simulink model "model_6DOF_V01"  (R2024b)
settings: Solver=VariableStepAuto  StartTime=0.0  StopTime=4  RelTol=1e-3
undefined symbols (not defined in the file or in its folder): p_RatGearFr_na, p_RatGearRe_na, p_RatSt_na, p_trackFr_m, p_trackRe_m, VEH
libraries: simulink x12, autolibutils x3, VUT_lib x3, sharedtransform x2, vehdynlibtire x2, CTRL x1, ESTS x1, INP x1, FUSI x1, OUT x1, vehdynlibeom x1, vehdynlibsuspension x1
(part 1 of 3)
settings Model: Creator=blatak  LastModifiedBy=jmbsp

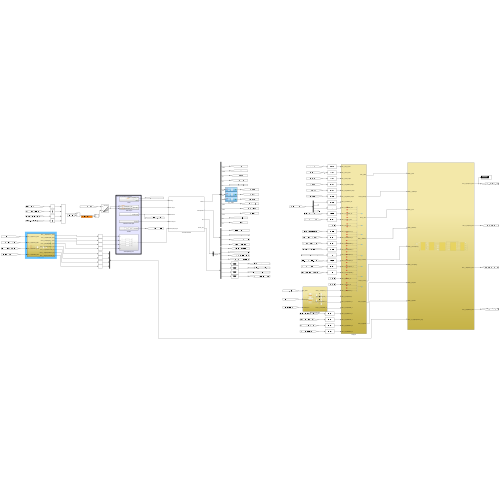
[thumbnail: Simulink's stored preview of the top-level diagram]
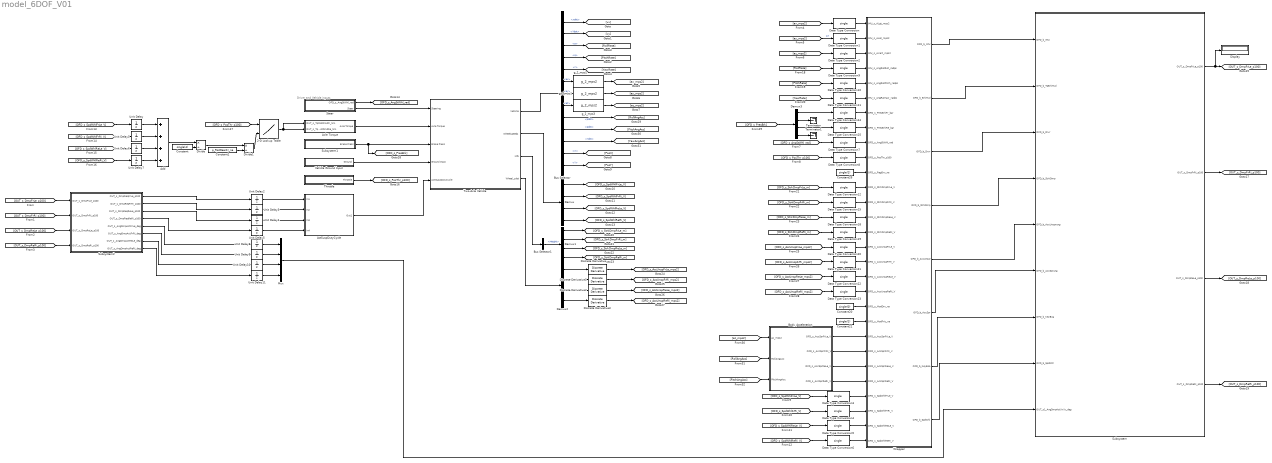
== system model_6DOF_V01 ==
  note: Driver and Vehicle inputs
  2-D Lookup Table : Lookup_n-D  BreakpointsForDimension1=[0 20 40 60 80 100]  BreakpointsForDimension2=[0 2000 4000 6000 8000 10000 12000]  Table=[0 0 0 0 0 0 0;200 200 200 200 150 100 50;350 350 350 250 200 150 100;500 500 500 350 250 150 150;650 650 650 450 350 250 200;800 800 800 600 500 400 300]  InternalRulePriority=Speed  RndMeth=Simplest
      settings: InputPortMap=u0,u1
  ActSuspDutyCycle : Subsystem
  Add : Sum  Inputs=++++
  Axle Torque : Subsystem
  Body_Acceleration : Subsystem
  Bus Selector : BusSelector  OutputSignals=Vehicle.BdyFrm.Cg.Vel.xdot,Vehicle.InertFrm.Cg.Vel.Ydot,Vehicle.BdyFrm.Cg.AngVel.p,Vehicle.BdyFrm.Cg.AngVel.q,Vehicle.BdyFrm.Cg.AngVel.r,Vehicle.BdyFrm.Cg.Acc.ax,Vehicle.BdyFrm.Cg.Acc.ay,Vehicle.BdyFrm.Cg.Acc.az,Vehicle.BdyFrm.Cg.AngAcc.pdot,Vehicle.BdyFrm.Cg.AngAcc.qdot,Vehicle.BdyFrm.Cg.AngAcc.rdot,Vehicle.InertFrm.Cg.Disp.X,Vehicle.InertFrm.Cg.Disp.Y
  Bus Selector1 : BusSelector  OutputSignals=Height
  Constant : Constant  Value=single(4)
  Constant1 : Constant  Value=p_RatGearFr_na
  Constant20 : Constant  Value=single(0)
  Constant21 : Constant  Value=single(1)
  Constant26 : Constant  Value=single(1)
  Data Type Conversion{,1..12,15,18..25} (22 alike) : DataTypeConversion  OutDataTypeStr=single  SaturateOnIntegerOverflow=off  RndMeth=Floor
  Demux{,1..3} (4 alike) : Demux
  Discrete Derivative{,1..3} (4 alike) : simulink/Discrete/Discrete Derivative  gainval=1.0  ICPrevScaledInput=0.0  OutMin=[]  OutMax=[]  OutDataType=fixdt(1, 16)  OutScaling=2^-10  DoSatur=off
  Display : Display
  Divide : Product  Inputs=*/
  Divide1 : Product  Inputs=*/
  Mux : Mux
  Steer : Subsystem
  Subsystem : Subsystem
  Subsystem1 : Subsystem
  Subsystem2 : Subsystem
  Terminator : Terminator
  Terminator1 : Terminator
  Throttle : Subsystem
  Two-Axle Vehicle : Subsystem
  Unit Delay{,1..11} (12 alike) : UnitDelay  SampleTime=-1  HasFrameUpgradeWarning=on
  Vehicle Ground Input : Subsystem  VariantControl=0
  Wrapper : Subsystem
  g_2_mps1 : VUT_lib/g_2_mps2  SystemSampleTime=-1  VariantActivationTime=update diagram  AllowFlexibleInterface=on  Latency=0  AutoFrameSizeCalculation=off
  g_2_mps2 : VUT_lib/g_2_mps2  SystemSampleTime=-1  VariantActivationTime=update diagram  AllowFlexibleInterface=on  Latency=0  AutoFrameSizeCalculation=off
  g_2_mps3 : VUT_lib/g_2_mps2  SystemSampleTime=-1  VariantActivationTime=update diagram  AllowFlexibleInterface=on  Latency=0  AutoFrameSizeCalculation=off
  wires:
  [OFD_s_AccUnspFrRi_mps2] -> Data Type Conversion21/1
  [OFD_s_AccUnspFrLe_mps2] -> Data Type Conversion20/1
  Data Type Conversion9/1 -> Wrapper/4(IMU_s_AngRatRoll_radps)
  Subsystem/1(OUT_s_DmpFrLe_p100) -> Display/1, [OUT_s_DmpFrLe_p100]
  Wrapper/7(OFD_b_KeyBoa) -> Subsystem/7(OFD_b_KeyBoa)
  Body_Acceleration/4(OFD_s_AccSprReRi_V) -> Wrapper/25(OFD_s_AccSprReRi_V)
  Body_Acceleration/1(OFD_s_AccSprFrLe_V) -> Wrapper/22(OFD_s_AccSprFrLe_V)
  Constant26/1 -> Wrapper/11(OFD_s_RegDrv_na)
  [ax_mps2] -> Data Type Conversion/1
  [OFD_s_AngStWhl_rad] -> Data Type Conversion7/1
  Body_Acceleration/2(OFD_s_AccSprFrRi_V) -> Wrapper/23(OFD_s_AccSprFrRi_V)
  Wrapper/1(OFD_b_IMU) -> Subsystem/1(OFD_b_IMU)
  [OFD_s_AccUnspReRi_mps2] -> Data Type Conversion23/1
  Constant20/1 -> Wrapper/20(OFD_s_ModDrv_na)
  [OFD_s_SpdWhlReRi_V] -> Data Type Conversion6/1
  Wrapper/8(OFD_b_SpdWhl) -> Subsystem/8(OFD_b_SpdWhl)
  Wrapper/4(OFD_b_StrkDmp) -> Subsystem/4(OFD_b_StrkDmp)
  Wrapper/2(OFD_b_BrkHyd) -> Subsystem/2(OFD_b_TqBrkHyd)
  [ay_mps2] -> Data Type Conversion1/1  "AY"
  [OFD_s_StrkDmpFrRi_m] -> Data Type Conversion15/1
  [OFD_s_StrkDmpReLe_m] -> Data Type Conversion18/1
  Wrapper/3(OFD_b_Drvr) -> Subsystem/3(OFD_b_Drvr)
  [OFD_s_AccUnspReLe_mps2] -> Data Type Conversion22/1
  [az_mps2] -> Data Type Conversion2/1
  Data Type Conversion10/1 -> Wrapper/5(IMU_s_AngRatPitch_radps)
  Wrapper/6(OFD_b_AccSpr) -> Subsystem/6(OFD_b_AccSprung)
  [OFD_s_SpdWhlReLe_V] -> Data Type Conversion5/1
  [OFD_s_StrkDmpReRi_m] -> Data Type Conversion19/1
  Demux3/1 -> Data Type Conversion24/1
  Subsystem/2(OUT_s_DmpFrRi_p100) -> [OUT_s_DmpFrRi_p100]
  Constant21/1 -> Wrapper/21(OFD_s_ModFric_na)
  [OFD_s_PosThr_p100] -> Data Type Conversion8/1
  Body_Acceleration/3(OFD_s_AccSprReLe_V) -> Wrapper/24(OFD_s_AccSprReLe_V)
  Wrapper/5(OFD_b_AccUnspr) -> Subsystem/5(OFD_b_AccUnsprung)
  Demux3/3 -> Data Type Conversion25/1
  [OFD_s_SpdWhlFrRi_V] -> Data Type Conversion4/1
  Data Type Conversion11/1 -> Wrapper/6(IMU_s_AngRatYaw_radps)
  [OFD_s_SpdWhlFrLe_V] -> Data Type Conversion3/1
  Subsystem/3(OUT_s_DmpReLe_p100) -> [OUT_s_DmpReLe_p100]
  g_2_mps2/1 -> [ax_mps2]
  Bus Selector/12 -> [PosX]  "<X>"
  Bus Selector/1 -> [vx]  "<xdot>"
  Throttle/1(Throttle) -> [OFD_s_PosThr_p100]
  Two-Axle Vehicle/1(Vehicle) -> Bus Selector/1
  Axle Torque/1(Axle Torque) -> Two-Axle Vehicle/2(Axle Torque)
  Bus Selector/13 -> [PosY]  "<Y>"
  Demux/2 -> [OFD_s_SpdWhlFrRi_V]
  Bus Selector/3 -> [RollRate]  "<p>"
  Demux/1 -> [OFD_s_SpdWhlFrLe_V]
  Bus Selector/5 -> [YawRate]  "<r>"
  g_2_mps1/1 -> [ay_mps2]
  Two-Axle Vehicle/2(Wheelspeeds) -> Demux/1
  2-D Lookup Table/1 -> Axle Torque/1(OUT_s_TqMotDmdFr_Nm), Axle Torque/2(OUT_s_TqMotDmdRe_Nm)
  Steer/1(OFD_s_AngStWhl_rad) -> [OFD_s_AngStWhl_rad]
  Vehicle Ground Input/1(Ground) -> Two-Axle Vehicle/4(Ground Input)
  Bus Selector/8 -> g_2_mps3/1  "<az>"
  g_2_mps3/1 -> [az_mps2]
  Bus Selector/6 -> g_2_mps2/1  "<ax>"
  Steer/2(Steer) -> Two-Axle Vehicle/1(Steering)
  Bus Selector/4 -> [PitchRate]  "<q>"
  Demux/3 -> [OFD_s_SpdWhlReLe_V]
  Demux/4 -> [OFD_s_SpdWhlReRi_V]
  Bus Selector/7 -> g_2_mps1/1  "<ay>"
  Bus Selector/2 -> [vy]  "<Ydot>"
  ActSuspDutyCycle/1(Out1) -> Two-Axle Vehicle/5(ActSuspDutyCycle)
  Unit Delay2/1 -> ActSuspDutyCycle/1(In1)
  Unit Delay3/1 -> ActSuspDutyCycle/2(In2)
  Unit Delay4/1 -> ActSuspDutyCycle/3(In3)
  Unit Delay5/1 -> ActSuspDutyCycle/4(In4)
  Subsystem/4(OUT_s_DmpReRi_p100) -> [OUT_s_DmpReRi_p100]
  Subsystem2/4(OUT_s_DmpReqReRi_p100) -> Unit Delay5/1
  Subsystem2/3(OUT_s_DmpReqReLe_p100) -> Unit Delay4/1
  Subsystem2/2(OUT_s_DmpReqFrRi_p100) -> Unit Delay3/1
  Subsystem2/1(OUT_s_DmpReqFrLe_p100) -> Unit Delay2/1
  Data Type Conversion/1 -> Wrapper/1(IMU_s_ALgt_mps2)
  Data Type Conversion1/1 -> Wrapper/2(IMU_s_ALat_mps2)
  Data Type Conversion2/1 -> Wrapper/3(IMU_s_AVert_mps2)
  Two-Axle Vehicle/3(Info) -> Bus Selector1/1
  Bus Selector1/1 -> Demux1/1  "<Height>"
  Data Type Conversion3/1 -> Wrapper/26(OFD_s_SpdWhlFrLe_V)
  Data Type Conversion4/1 -> Wrapper/27(OFD_s_SpdWhlFrRi_V)
  Data Type Conversion5/1 -> Wrapper/28(OFD_s_SpdWhlReLe_V)
  Data Type Conversion6/1 -> Wrapper/29(OFD_s_SpdWhlReRi_V)
  Data Type Conversion7/1 -> Wrapper/9(OFD_s_AngStWhl_rad)
  Data Type Conversion8/1 -> Wrapper/10(OFD_s_PosThr_p100)
  [OFD_s_SpdWhlFrLe_V] -> Unit Delay/1
  [OFD_s_SpdWhlFrRi_V] -> Unit Delay1/1
  [OFD_s_SpdWhlReLe_V] -> Unit Delay6/1
  [OFD_s_SpdWhlReRi_V] -> Unit Delay7/1
  Add/1 -> Divide/1
  Constant/1 -> Divide/2
  Divide/1 -> Divide1/1
  Constant1/1 -> Divide1/2
  Divide1/1 -> 2-D Lookup Table/2
  [OFD_s_PosThr_p100] -> 2-D Lookup Table/1
  Unit Delay/1 -> Add/1
  Unit Delay1/1 -> Add/2
  Unit Delay6/1 -> Add/3
  Unit Delay7/1 -> Add/4
  [RollRate] -> Data Type Conversion9/1
  [PitchRate] -> Data Type Conversion10/1
  [YawRate] -> Data Type Conversion11/1
  Demux1/1 -> [OFD_s_StrkDmpFrLe_m]
  Demux1/4 -> [OFD_s_StrkDmpReRi_m]
  Demux1/3 -> [OFD_s_StrkDmpReLe_m]
  Demux1/2 -> [OFD_s_StrkDmpFrRi_m]
  [OFD_s_StrkDmpFrLe_m] -> Data Type Conversion12/1
  Data Type Conversion12/1 -> Wrapper/12(OFD_s_StrkDmpFrLe_V)
  Data Type Conversion15/1 -> Wrapper/13(OFD_s_StrkDmpFrRi_V)
  Data Type Conversion18/1 -> Wrapper/14(OFD_s_StrkDmpReLe_V)
  Data Type Conversion19/1 -> Wrapper/15(OFD_s_StrkDmpReRi_V)
  Two-Axle Vehicle/4(Wheel_zdot) -> Demux2/1
  Demux2/1 -> Discrete Derivative/1
  Demux2/4 -> Discrete Derivative3/1
  Demux2/3 -> Discrete Derivative2/1
  Demux2/2 -> Discrete Derivative1/1
  Data Type Conversion20/1 -> Wrapper/16(OFD_s_AccUnspFrLe_V)
  Data Type Conversion21/1 -> Wrapper/17(OFD_s_AccUnspFrRi_V)
  Data Type Conversion22/1 -> Wrapper/18(OFD_s_AccUnspReLe_V)
  Data Type Conversion23/1 -> Wrapper/19(OFD_s_AccUnspReRi_V)
  [OFD_s_PresBrk] -> Demux3/1
  Demux3/2 -> Terminator/1
  Demux3/4 -> Terminator1/1
  Data Type Conversion24/1 -> Wrapper/7(OFD_s_PresBrkFr_bar)
  Data Type Conversion25/1 -> Wrapper/8(OFD_s_PresBrkRe_bar)
  Subsystem1/1(Brake Press) -> [OFD_s_PresBrk], Two-Axle Vehicle/3(Brake Press)
  Discrete Derivative/1 -> [OFD_s_AccUnspFrLe_mps2]
  Discrete Derivative1/1 -> [OFD_s_AccUnspFrRi_mps2]
  Discrete Derivative2/1 -> [OFD_s_AccUnspReLe_mps2]
  Discrete Derivative3/1 -> [OFD_s_AccUnspReRi_mps2]
  Bus Selector/9 -> [RollAngAcc]  "<pdot>"
  Bus Selector/10 -> [PitchAngAcc]  "<qdot>"
  Bus Selector/11 -> [YawAngAcc]  "<rdot>"
  [az_mps2] -> Body_Acceleration/1(az_mps2)
  [RollAngAcc] -> Body_Acceleration/2(RollAngAcc)
  [PitchAngAcc] -> Body_Acceleration/3(PitchAngAcc)
  [OUT_s_DmpFrLe_p100] -> Subsystem2/1(OUT_s_DmpFrLe_p100)
  [OUT_s_DmpFrRi_p100] -> Subsystem2/2(OUT_s_DmpFrRi_p100)
  [OUT_s_DmpReLe_p100] -> Subsystem2/3(OUT_s_DmpReLe_p100)
  [OUT_s_DmpReRi_p100] -> Subsystem2/4(OUT_s_DmpReRi_p100)
  Subsystem2/5(OUT_s_AngDmpActFrLe_deg) -> Unit Delay8/1
  Subsystem2/6(OUT_s_AngDmpActFrRi_deg) -> Unit Delay9/1
  Subsystem2/7(OUT_s_AngDmpActReLe_deg) -> Unit Delay10/1
  Subsystem2/8(OUT_s_AngDmpActReRi_deg) -> Unit Delay11/1
  Unit Delay11/1 -> Mux/4
  Unit Delay10/1 -> Mux/3
  Unit Delay9/1 -> Mux/2
  Unit Delay8/1 -> Mux/1
  Mux/1 -> Subsystem/9(OUT_s1_AngDmpActXxYy_deg)

== system model_6DOF_V01/ActSuspDutyCycle ==
  In1 : Inport
  In2 : Inport  Port=2
  In3 : Inport  Port=3
  In4 : Inport  Port=4
  Data Type Conversion{,1..3} (4 alike) : DataTypeConversion  OutDataTypeStr=double  SaturateOnIntegerOverflow=off  RndMeth=Floor
  Mux : Mux
  Out1 : Outport
  wires:
  Mux/1 -> Out1/1
  In1/1 -> Data Type Conversion/1
  Data Type Conversion/1 -> Mux/1
  In2/1 -> Data Type Conversion1/1
  Data Type Conversion1/1 -> Mux/2
  In3/1 -> Data Type Conversion2/1
  Data Type Conversion2/1 -> Mux/3
  In4/1 -> Data Type Conversion3/1
  Data Type Conversion3/1 -> Mux/4

== system model_6DOF_V01/Axle Torque ==
  OUT_s_TqMotDmdFr_Nm : Inport
  OUT_s_TqMotDmdRe_Nm : Inport  Port=2
  Constant1 : Constant  Value=p_RatGearRe_na
  Constant12 : Constant  Value=single(2)
  Constant2 : Constant  Value=single(2)
  Constant3 : Constant  Value=p_RatGearFr_na
  Data Type Conversion{,1..3} (4 alike) : DataTypeConversion  OutDataTypeStr=double  SaturateOnIntegerOverflow=off  RndMeth=Floor
  Divide : Product  Inputs=*/
  Divide1 : Product  Inputs=*/
  Mux : Mux
  Product : Product
  Product1 : Product
  Axle Torque : Outport
  wires:
  Mux/1 -> Axle Torque/1
  OUT_s_TqMotDmdFr_Nm/1 -> Product/2
  OUT_s_TqMotDmdRe_Nm/1 -> Product1/1
  Constant3/1 -> Product/1
  Constant1/1 -> Product1/2
  Product/1 -> Divide/1
  Constant12/1 -> Divide/2
  Product1/1 -> Divide1/1
  Constant2/1 -> Divide1/2
  Divide/1 -> Data Type Conversion1/1, Data Type Conversion/1
  Data Type Conversion/1 -> Mux/1
  Data Type Conversion1/1 -> Mux/2
  Data Type Conversion3/1 -> Mux/4
  Data Type Conversion2/1 -> Mux/3
  Divide1/1 -> Data Type Conversion3/1, Data Type Conversion2/1

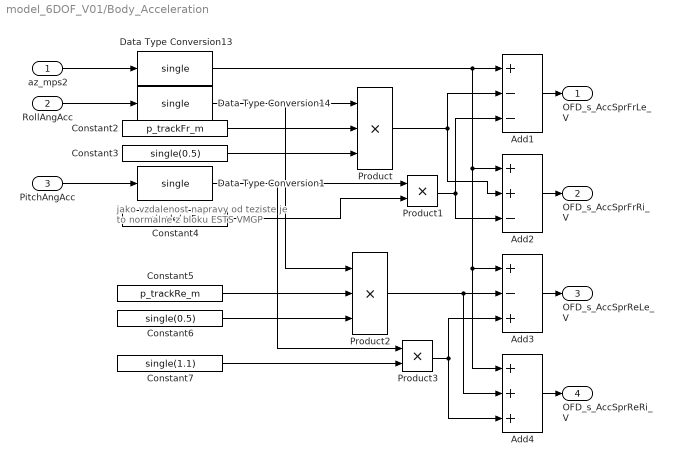
== system model_6DOF_V01/Body_Acceleration ==
  note: jako vzdalenost napravy od teziste
      | je to normalne z bloku ESTS VMGP
  az_mps2 : Inport
  RollAngAcc : Inport  Port=2
  PitchAngAcc : Inport  Port=3
  Add1 : Sum  Inputs=+--
  Add2 : Sum  Inputs=++-
  Add3 : Sum  Inputs=+-+
  Add4 : Sum  Inputs=+++
  Constant2 : Constant  Value=p_trackFr_m
  Constant3 : Constant  Value=single(0.5)
  Constant4 : Constant  Value=single(1.5)
  Constant5 : Constant  Value=p_trackRe_m
  Constant6 : Constant  Value=single(0.5)
  Constant7 : Constant  Value=single(1.1)
  Data Type Conversion1 : DataTypeConversion  OutDataTypeStr=single  SaturateOnIntegerOverflow=off  RndMeth=Floor
  Data Type Conversion13 : DataTypeConversion  OutDataTypeStr=single  SaturateOnIntegerOverflow=off  RndMeth=Floor
  Data Type Conversion14 : DataTypeConversion  OutDataTypeStr=single  SaturateOnIntegerOverflow=off  RndMeth=Floor
  Product : Product  Inputs=3
  Product1 : Product
  Product2 : Product  Inputs=3
  Product3 : Product
  OFD_s_AccSprFrLe_V : Outport
  OFD_s_AccSprFrRi_V : Outport  Port=2
  OFD_s_AccSprReLe_V : Outport  Port=3
  OFD_s_AccSprReRi_V : Outport  Port=4
  wires:
  Add3/1 -> OFD_s_AccSprReLe_V/1
  PitchAngAcc/1 -> Data Type Conversion1/1
  Product1/1 -> Add1/3, Add2/3
  Add1/1 -> OFD_s_AccSprFrLe_V/1
  Product2/1 -> Add4/2, Add3/2
  Data Type Conversion13/1 -> Add1/1, Add4/1, Add3/1, Add2/1
  Constant4/1 -> Product1/2
  Product/1 -> Add1/2, Add2/2
  Constant3/1 -> Product/3
  Constant7/1 -> Product3/2
  az_mps2/1 -> Data Type Conversion13/1
  Constant5/1 -> Product2/2
  Constant2/1 -> Product/2
  Product3/1 -> Add3/3, Add4/3
  Constant6/1 -> Product2/3
  Add4/1 -> OFD_s_AccSprReRi_V/1
  Add2/1 -> OFD_s_AccSprFrRi_V/1
  RollAngAcc/1 -> Data Type Conversion14/1
  Data Type Conversion1/1 -> Product3/1, Product1/1
  Data Type Conversion14/1 -> Product2/1, Product/1

== system model_6DOF_V01/Steer ==
  Constant22 : Constant  Value=p_RatSt_na
  Divide : Product  Inputs=*/
  Mux : Mux  Inputs=2
  Ramp : simulink/Sources/Ramp  slope=0.5  start=2  InitialOutput=0
  Saturation : Saturate  UpperLimit=1  LowerLimit=-1
  OFD_s_AngStWhl_rad : Outport
  Steer : Outport  Port=2
  wires:
  Mux/1 -> Steer/1
  Saturation/1 -> OFD_s_AngStWhl_rad/1, Divide/1
  Constant22/1 -> Divide/2
  Divide/1 -> Mux/2, Mux/1  "WhlStAng"
  Ramp/1 -> Saturation/1

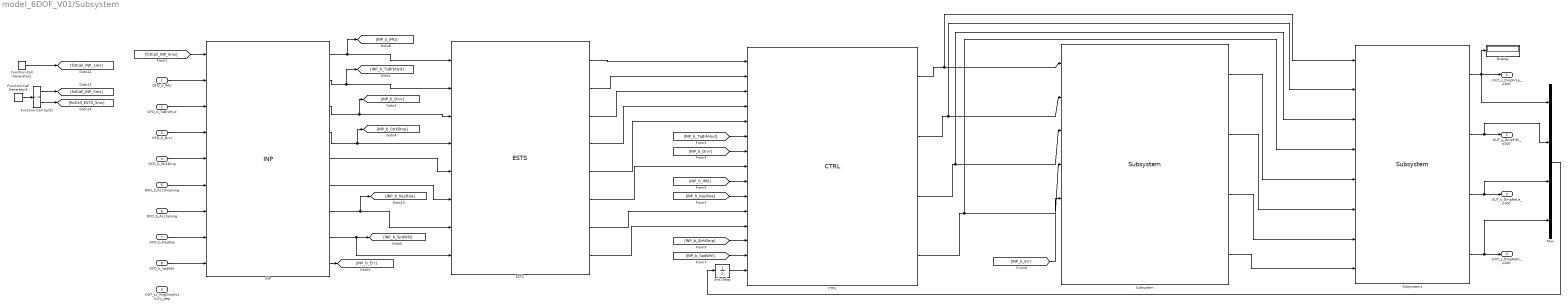
== system model_6DOF_V01/Subsystem ==
  OFD_b_IMU : Inport
  OFD_b_TqBrkHyd : Inport  Port=2
  OFD_b_Drvr : Inport  Port=3
  OFD_b_StrkDmp : Inport  Port=4
  OFD_b_AccUnsprung : Inport  Port=5
  OFD_b_AccSprung : Inport  Port=6
  OFD_b_KeyBoa : Inport  Port=7
  OFD_b_SpdWhl : Inport  Port=8
  OUT_s1_AngDmpActXxYy_deg : Inport  Port=9
  CTRL : CTRL/CTRL  SystemSampleTime=-1  VariantActivationTime=update diagram  AllowFlexibleInterface=on  Latency=0  AutoFrameSizeCalculation=off
  Display : Display
  ESTS : ESTS/ESTS  SystemSampleTime=-1  VariantActivationTime=update diagram  AllowFlexibleInterface=on  Latency=0  AutoFrameSizeCalculation=off
  Function-Call Generator2 : simulink/Ports & Subsystems/Function-Call Generator  sample_time=1  numberOfIterations=1  DisallowWideOutput=off
  Function-Call Generator3 : simulink/Ports & Subsystems/Function-Call Generator  sample_time=0.005  numberOfIterations=1  DisallowWideOutput=off
  Function-Call Split1 : FunctionCallSplit  IconShape=distinctive  NumOutputPorts=2  OutputPortLayout=default
  INP : INP/INP  SystemSampleTime=-1  VariantActivationTime=update diagram  AllowFlexibleInterface=on  Latency=0  AutoFrameSizeCalculation=off
      link override Function-Call Subsystem1/Bus Selector2: OutputSignals=OFD_s_AngStWhl_rad,OFD_s_PosThr_p100,OFD_s_RegDrv_na
  Mux : Mux
  Subsystem : FUSI/Subsystem  SystemSampleTime=-1  VariantActivationTime=update diagram  AllowFlexibleInterface=on  Latency=0  AutoFrameSizeCalculation=off
  Subsystem1 : OUT/Subsystem  SystemSampleTime=-1  VariantActivationTime=update diagram  AllowFlexibleInterface=on  Latency=0  AutoFrameSizeCalculation=off
  Unit Delay : UnitDelay  SampleTime=-1  HasFrameUpgradeWarning=on
  OUT_s_DmpFrLe_p100 : Outport
  OUT_s_DmpFrRi_p100 : Outport  Port=2
  OUT_s_DmpReLe_p100 : Outport  Port=3
  OUT_s_DmpReRi_p100 : Outport  Port=4
  wires:
  OFD_b_IMU/1 -> INP/2
  [fctCall_INP_5ms] -> INP/1
  OFD_b_Drvr/1 -> INP/4
  INP/3 -> [INP_b_Drvr], ESTS/3
  Function-Call Generator2/1 -> [fctCall_INP_1ms]
  Function-Call Generator3/1 -> Function-Call Split1/1
  INP/1 -> ESTS/1, [INP_b_IMU]
  Function-Call Split1/1 -> [fctCall_INP_5ms]
  Function-Call Split1/2 -> [fctCall_ESTS_5ms]
  ESTS/7 -> CTRL/11
  [INP_b_KeyBoa] -> CTRL/10
  [INP_b_Drvr] -> CTRL/7
  [INP_b_TqBrkHyd] -> CTRL/6
  ESTS/6 -> CTRL/8
  [INP_b_IMU] -> CTRL/9
  CTRL/1 -> Subsystem1/1, Subsystem/1
  CTRL/2 -> Subsystem1/2, Subsystem/2
  CTRL/3 -> Subsystem1/3, Subsystem/3
  CTRL/4 -> Subsystem1/4, Subsystem/4
  Subsystem1/1 -> Display/1, Mux/1, OUT_s_DmpFrLe_p100/1
  Subsystem1/2 -> Mux/2, OUT_s_DmpFrRi_p100/1
  Subsystem1/3 -> Mux/3, OUT_s_DmpReLe_p100/1
  Subsystem1/4 -> Mux/4, OUT_s_DmpReRi_p100/1
  [INP_b_StrkDmp] -> CTRL/13
  OFD_b_TqBrkHyd/1 -> INP/3
  OFD_b_StrkDmp/1 -> INP/5
  OFD_b_AccUnsprung/1 -> INP/6
  OFD_b_AccSprung/1 -> INP/7
  OFD_b_KeyBoa/1 -> INP/8
  INP/2 -> ESTS/2, [INP_b_TqBrkHyd]
  INP/4 -> [INP_b_StrkDmp], ESTS/4
  INP/5 -> ESTS/5
  INP/6 -> ESTS/6
  INP/7 -> ESTS/7, [INP_b_KeyBoa]
  ESTS/1 -> CTRL/1
  ESTS/2 -> CTRL/2
  ESTS/3 -> CTRL/3
  ESTS/4 -> CTRL/4
  ESTS/5 -> CTRL/5
  ESTS/8 -> CTRL/12
  [INP_b_Err] -> Subsystem/5
  Subsystem/1 -> Subsystem1/5
  Subsystem/2 -> Subsystem1/6
  Subsystem/3 -> Subsystem1/7
  Subsystem/4 -> Subsystem1/8
  OFD_b_SpdWhl/1 -> INP/9
  INP/8 -> [INP_b_SpdWhl], ESTS/8
  INP/9 -> [INP_b_Err]
  [INP_b_SpdWhl] -> CTRL/14
  Mux/1 -> Unit Delay/1
  Unit Delay/1 -> CTRL/15

== system model_6DOF_V01/Subsystem1 ==
  Mux : Mux
  Ramp : simulink/Sources/Ramp  slope=0  start=0  InitialOutput=0
  Saturation : Saturate
  Brake Press : Outport
  wires:
  Saturation/1 -> Mux/4, Mux/3, Mux/2, Mux/1
  Ramp/1 -> Saturation/1
  Mux/1 -> Brake Press/1

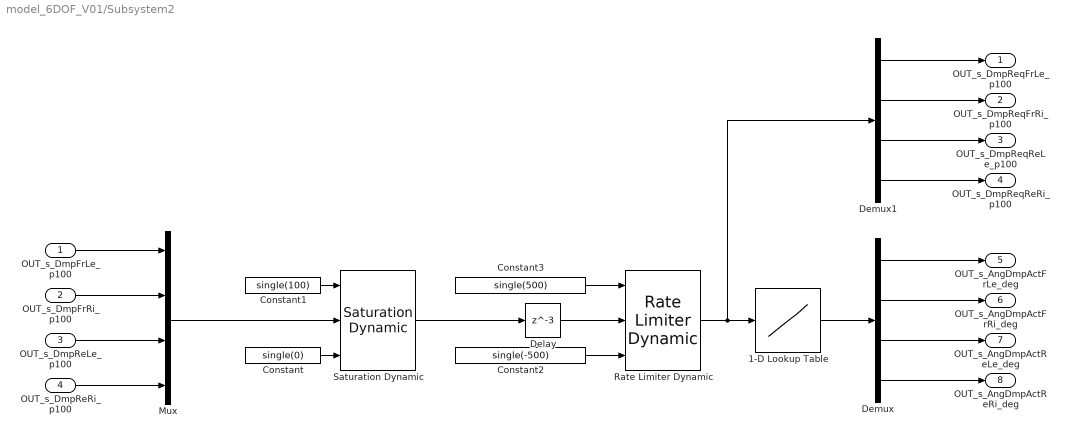
== system model_6DOF_V01/Subsystem2 ==
  OUT_s_DmpFrLe_p100 : Inport
  OUT_s_DmpFrRi_p100 : Inport  Port=2
  OUT_s_DmpReLe_p100 : Inport  Port=3
  OUT_s_DmpReRi_p100 : Inport  Port=4
  1-D Lookup Table : Lookup_n-D  NumberOfTableDimensions=1  BreakpointsForDimension1=[0 10 20 30 40 50 60 70 80 90 100]  Table=[0 5 10 15 20 25 30 35 40 45 50]  InternalRulePriority=Speed  RndMeth=Simplest
  Constant : Constant  Value=single(0)
  Constant1 : Constant  Value=single(100)
  Constant2 : Constant  Value=single(-500)
  Constant3 : Constant  Value=single(500)
  Delay : Delay  DelayLength=3
  Demux : Demux
  Demux1 : Demux
  Mux : Mux
  Rate Limiter Dynamic : simulink/Discontinuities/Rate Limiter Dynamic
  Saturation Dynamic : simulink/Discontinuities/Saturation Dynamic  OutMin=[]  OutMax=[]  OutDataTypeStr=Inherit: Same as second input  OutDataType=fixdt(1, 16)  OutScaling=2^-10  DoSatur=off
  OUT_s_DmpReqFrLe_p100 : Outport
  OUT_s_DmpReqFrRi_p100 : Outport  Port=2
  OUT_s_DmpReqReLe_p100 : Outport  Port=3
  OUT_s_DmpReqReRi_p100 : Outport  Port=4
  OUT_s_AngDmpActFrLe_deg : Outport  Port=5
  OUT_s_AngDmpActFrRi_deg : Outport  Port=6
  OUT_s_AngDmpActReLe_deg : Outport  Port=7
  OUT_s_AngDmpActReRi_deg : Outport  Port=8
  wires:
  OUT_s_DmpReRi_p100/1 -> Mux/4
  OUT_s_DmpReLe_p100/1 -> Mux/3
  OUT_s_DmpFrRi_p100/1 -> Mux/2
  OUT_s_DmpFrLe_p100/1 -> Mux/1
  Mux/1 -> Saturation Dynamic/2
  Constant/1 -> Saturation Dynamic/3
  Constant1/1 -> Saturation Dynamic/1
  Saturation Dynamic/1 -> Delay/1
  Delay/1 -> Rate Limiter Dynamic/2
  Constant2/1 -> Rate Limiter Dynamic/3
  Constant3/1 -> Rate Limiter Dynamic/1
  Rate Limiter Dynamic/1 -> Demux1/1, 1-D Lookup Table/1
  1-D Lookup Table/1 -> Demux/1
  Demux1/1 -> OUT_s_DmpReqFrLe_p100/1
  Demux1/2 -> OUT_s_DmpReqFrRi_p100/1
  Demux1/3 -> OUT_s_DmpReqReLe_p100/1
  Demux1/4 -> OUT_s_DmpReqReRi_p100/1
  Demux/1 -> OUT_s_AngDmpActFrLe_deg/1
  Demux/2 -> OUT_s_AngDmpActFrRi_deg/1
  Demux/3 -> OUT_s_AngDmpActReLe_deg/1
  Demux/4 -> OUT_s_AngDmpActReRi_deg/1

== system model_6DOF_V01/Throttle ==
  Ramp : simulink/Sources/Ramp  slope=10  start=3  InitialOutput=0
  Saturation : Saturate  UpperLimit=100  LowerLimit=0
  Throttle : Outport
  wires:
  Ramp/1 -> Saturation/1
  Saturation/1 -> Throttle/1

== system model_6DOF_V01/Two-Axle Vehicle ==
  Steering : Inport
  Axle Torque : Inport  Port=2
  Brake Press : Inport  Port=3
  Ground Input : Inport  Port=4
  ActSuspDutyCycle : Inport  Port=5
  Bus Creator : BusCreator  Inputs=2
  Bus Selector : BusSelector  OutputSignals=z,mu
  Bus Selector3 : BusSelector  OutputSignals=TireFrame.Omega,TireFrame.zdot
  Subsystem : Subsystem
  Vehicle Suspension : Subsystem
      mask Display: image('suspsacoil.png')
  Wheels and Tires : Subsystem
      mask Display: image('wheel3dof.png')
  Vehicle : Outport
  Wheelspeeds : Outport  Port=2
  Info : Outport  Port=3
  Wheel_zdot : Outport  Port=4
  wires:
  Bus Selector/1 -> Wheels and Tires/4(Ground Input)  "<z>"
  Vehicle Suspension/1(Suspension) -> Bus Creator/2, Subsystem/1(Suspension), Wheels and Tires/1(Suspension)  "Suspension"
  Subsystem/1(Vehicle1) -> Bus Creator/1, Vehicle Suspension/3(Vehicle)  "Vehicle"
  Wheels and Tires/1(Wheels) -> Vehicle Suspension/2(Wheels), Bus Selector3/1  "Wheels"
  Bus Selector/2 -> Wheels and Tires/5(Friction)  "<mu>"
  Axle Torque/1 -> Wheels and Tires/2(Axle Torque)
  Steering/1 -> Vehicle Suspension/1(Steering)
  Brake Press/1 -> Wheels and Tires/3(Brake Press)
  Ground Input/1 -> Bus Selector/1
  Bus Creator/1 -> Vehicle/1
  Bus Selector3/1 -> Wheelspeeds/1  "<Omega>"
  ActSuspDutyCycle/1 -> Vehicle Suspension/4(ActSuspDutyCycle)
  Vehicle Suspension/2(Info) -> Info/1
  Bus Selector3/2 -> Wheel_zdot/1  "<zdot>"

== system model_6DOF_V01/Vehicle Ground Input ==
  Bus Creator : BusCreator  Inputs=4
  Bus Creator2 : BusCreator  Inputs=4
  Bus Creator3 : BusCreator  Inputs=2
  Constant1 : Constant  Value=zeros(4,1)
  Demux : Demux
  Demux1 : Demux
  Friction : Constant  Value=ones(4,1).*1.0
  Signal Specification : SignalSpecification  Unit=m
  Signal Specification1 : SignalSpecification  Unit=1
  Ground : Outport  VectorParamsAs1DForOutWhenUnconnected=off
  wires:
  Bus Creator3/1 -> Ground/1
  Signal Specification1/1 -> Demux1/1
  Friction/1 -> Signal Specification1/1
  Bus Creator2/1 -> Bus Creator3/2  "mu"
  Bus Creator/1 -> Bus Creator3/1  "z"
  Demux/2 -> Bus Creator/2  "G_FR_z"
  Demux/3 -> Bus Creator/3  "G_RL_z"
  Demux/1 -> Bus Creator/1  "G_FL_z"
  Demux/4 -> Bus Creator/4  "G_RR_z"
  Signal Specification/1 -> Demux/1
  Constant1/1 -> Signal Specification/1
  Demux1/2 -> Bus Creator2/2  "mu_FR"
  Demux1/1 -> Bus Creator2/1  "mu_FL"
  Demux1/3 -> Bus Creator2/3  "mu_RL"
  Demux1/4 -> Bus Creator2/4  "mu_RR"

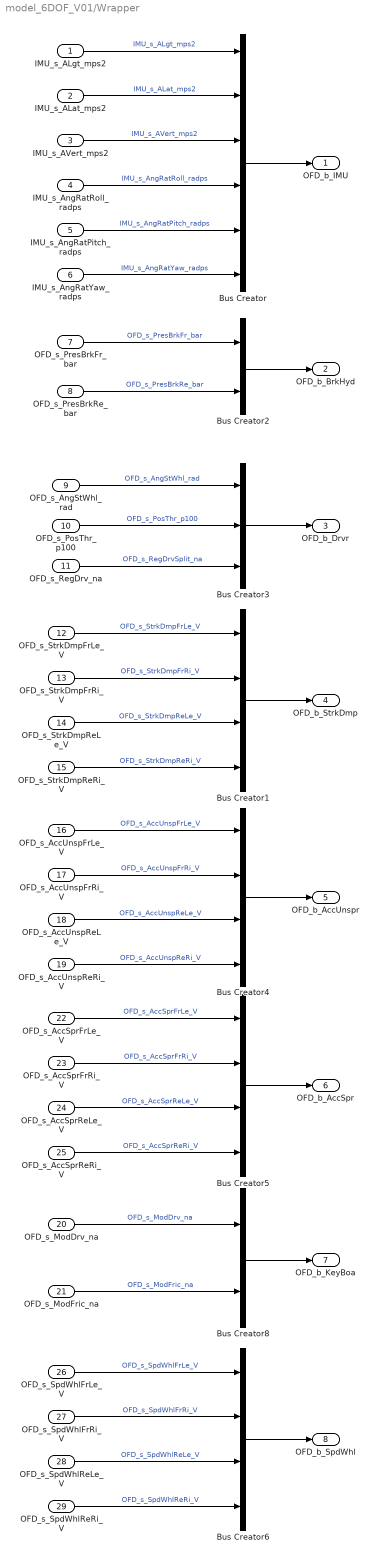
== system model_6DOF_V01/Wrapper ==
  IMU_s_ALgt_mps2 : Inport
  IMU_s_ALat_mps2 : Inport  Port=2
  IMU_s_AVert_mps2 : Inport  Port=3
  IMU_s_AngRatRoll_radps : Inport  Port=4
  IMU_s_AngRatPitch_radps : Inport  Port=5
  IMU_s_AngRatYaw_radps : Inport  Port=6
  OFD_s_PresBrkFr_bar : Inport  Port=7
  OFD_s_PresBrkRe_bar : Inport  Port=8
  OFD_s_AngStWhl_rad : Inport  Port=9
  OFD_s_PosThr_p100 : Inport  Port=10
  OFD_s_RegDrv_na : Inport  Port=11
  OFD_s_StrkDmpFrLe_V : Inport  Port=12
  OFD_s_StrkDmpFrRi_V : Inport  Port=13
  OFD_s_StrkDmpReLe_V : Inport  Port=14
  OFD_s_StrkDmpReRi_V : Inport  Port=15
  OFD_s_AccUnspFrLe_V : Inport  Port=16
  OFD_s_AccUnspFrRi_V : Inport  Port=17
  OFD_s_AccUnspReLe_V : Inport  Port=18
  OFD_s_AccUnspReRi_V : Inport  Port=19
  OFD_s_ModDrv_na : Inport  Port=20
  OFD_s_ModFric_na : Inport  Port=21
  OFD_s_AccSprFrLe_V : Inport  Port=22
  OFD_s_AccSprFrRi_V : Inport  Port=23
  OFD_s_AccSprReLe_V : Inport  Port=24
  OFD_s_AccSprReRi_V : Inport  Port=25
  OFD_s_SpdWhlFrLe_V : Inport  Port=26
  OFD_s_SpdWhlFrRi_V : Inport  Port=27
  OFD_s_SpdWhlReLe_V : Inport  Port=28
  OFD_s_SpdWhlReRi_V : Inport  Port=29
  Bus Creator : BusCreator  Inputs=6  OutDataTypeStr=Bus: OFD_b_IMU
      settings: InheritFromInputs=off
  Bus Creator1 : BusCreator  Inputs=4  OutDataTypeStr=Bus: OFD_b_StrkDmp
      settings: InheritFromInputs=off
  Bus Creator2 : BusCreator  Inputs=2  OutDataTypeStr=Bus: OFD_b_TqBrkHyd
      settings: InheritFromInputs=off
  Bus Creator3 : BusCreator  Inputs=3  OutDataTypeStr=Bus: OFD_b_Drvr
      settings: InheritFromInputs=off
  Bus Creator4 : BusCreator  Inputs=4  OutDataTypeStr=Bus: OFD_b_AccUnsp
      settings: InheritFromInputs=off
  Bus Creator5 : BusCreator  Inputs=4  OutDataTypeStr=Bus: OFD_b_AccSpr
      settings: InheritFromInputs=off
  Bus Creator6 : BusCreator  Inputs=4  OutDataTypeStr=Bus: OFD_b_SpdWhl
      settings: InheritFromInputs=off
  Bus Creator8 : BusCreator  Inputs=2  OutDataTypeStr=Bus: OFD_b_KeyBoa
      settings: InheritFromInputs=off
  OFD_b_IMU : Outport
  OFD_b_BrkHyd : Outport  Port=2
  OFD_b_Drvr : Outport  Port=3
  OFD_b_StrkDmp : Outport  Port=4
  OFD_b_AccUnspr : Outport  Port=5
  OFD_b_AccSpr : Outport  Port=6
  OFD_b_KeyBoa : Outport  Port=7
  OFD_b_SpdWhl : Outport  Port=8
  wires:
  IMU_s_ALgt_mps2/1 -> Bus Creator/1  "IMU_s_ALgt_mps2"
  IMU_s_AngRatYaw_radps/1 -> Bus Creator/6  "IMU_s_AngRatYaw_radps"
  IMU_s_AngRatPitch_radps/1 -> Bus Creator/5  "IMU_s_AngRatPitch_radps"
  IMU_s_AngRatRoll_radps/1 -> Bus Creator/4  "IMU_s_AngRatRoll_radps"
  IMU_s_AVert_mps2/1 -> Bus Creator/3  "IMU_s_AVert_mps2"
  IMU_s_ALat_mps2/1 -> Bus Creator/2  "IMU_s_ALat_mps2"
  Bus Creator/1 -> OFD_b_IMU/1
  OFD_s_PresBrkFr_bar/1 -> Bus Creator2/1  "OFD_s_PresBrkFr_bar"
  OFD_s_PresBrkRe_bar/1 -> Bus Creator2/2  "OFD_s_PresBrkRe_bar"
  Bus Creator2/1 -> OFD_b_BrkHyd/1
  OFD_s_AngStWhl_rad/1 -> Bus Creator3/1  "OFD_s_AngStWhl_rad"
  OFD_s_PosThr_p100/1 -> Bus Creator3/2  "OFD_s_PosThr_p100"
  OFD_s_AccUnspFrLe_V/1 -> Bus Creator4/1  "OFD_s_AccUnspFrLe_V"
  OFD_s_AccUnspFrRi_V/1 -> Bus Creator4/2  "OFD_s_AccUnspFrRi_V"
  OFD_s_StrkDmpFrRi_V/1 -> Bus Creator1/2  "OFD_s_StrkDmpFrRi_V"
  OFD_s_StrkDmpFrLe_V/1 -> Bus Creator1/1  "OFD_s_StrkDmpFrLe_V"
  Bus Creator3/1 -> OFD_b_Drvr/1
  Bus Creator4/1 -> OFD_b_AccUnspr/1
  OFD_s_ModFric_na/1 -> Bus Creator8/2  "OFD_s_ModFric_na"
  OFD_s_ModDrv_na/1 -> Bus Creator8/1  "OFD_s_ModDrv_na"
  Bus Creator8/1 -> OFD_b_KeyBoa/1
  OFD_s_RegDrv_na/1 -> Bus Creator3/3  "OFD_s_RegDrvSplit_na"
  OFD_s_AccUnspReLe_V/1 -> Bus Creator4/3  "OFD_s_AccUnspReLe_V"
  OFD_s_AccUnspReRi_V/1 -> Bus Creator4/4  "OFD_s_AccUnspReRi_V"
  OFD_s_AccSprReRi_V/1 -> Bus Creator5/4  "OFD_s_AccSprReRi_V"
  OFD_s_AccSprFrRi_V/1 -> Bus Creator5/2  "OFD_s_AccSprFrRi_V"
  OFD_s_AccSprReLe_V/1 -> Bus Creator5/3  "OFD_s_AccSprReLe_V"
  OFD_s_AccSprFrLe_V/1 -> Bus Creator5/1  "OFD_s_AccSprFrLe_V"
  OFD_s_StrkDmpReLe_V/1 -> Bus Creator1/3  "OFD_s_StrkDmpReLe_V"
  OFD_s_StrkDmpReRi_V/1 -> Bus Creator1/4  "OFD_s_StrkDmpReRi_V"
  Bus Creator1/1 -> OFD_b_StrkDmp/1
  Bus Creator5/1 -> OFD_b_AccSpr/1
  OFD_s_SpdWhlFrLe_V/1 -> Bus Creator6/1  "OFD_s_SpdWhlFrLe_V"
  OFD_s_SpdWhlFrRi_V/1 -> Bus Creator6/2  "OFD_s_SpdWhlFrRi_V"
  Bus Creator6/1 -> OFD_b_SpdWhl/1
  OFD_s_SpdWhlReLe_V/1 -> Bus Creator6/3  "OFD_s_SpdWhlReLe_V"
  OFD_s_SpdWhlReRi_V/1 -> Bus Creator6/4  "OFD_s_SpdWhlReRi_V"

== system model_6DOF_V01/Two-Axle Vehicle/Subsystem ==
  Suspension : Inport
  Bus Selector3 : BusSelector  OutputSignals=Veh.F,Veh.M
  Constant : Constant  Value=zeros(3,1)
  Ground : Ground
  Ground1 : Ground
  Terminator{6..11} (6 alike) : Terminator
  Vehicle Body 6DOF : vehdynlibeom/Vehicle Body 6DOF  extPos=on  extVel=on  extEuler=on  extRotRate=on  htchFMode=off  htchMMode=off  m=VEH.Mass  a=VEH.FrontAxlePositionfromCG  b=VEH.RearAxlePositionfromCG  d=0  h=VEH.HeightCG  dh=VEH.HitchDistance  hl=0  hh=VEH.HitchHeight  Xe_o=[VEH.InitialLongPosition,VEH.InitialLatPosition,VEH.InitialVertPosition]  xbdot_o=[VEH.InitialLongVel,VEH.InitialLatVel,VEH.InitialVertVel]  eul_o=[VEH.InitialRollAngle,VEH.InitialPitchAngle,VEH.InitialYawAngle]  p_o=[VEH.InitialRollRate,VEH.InitialPitchRate,VEH.InitialYawRate]  Iveh=[VEH.RollMomentInertia 0 0; 0 VEH.PitchMomentInertia 0; 0 0 VEH.YawMomentInertia]  w=VEH.TrackWidth.*[1 1]  z1m=0  z1R=[-.25,.125,.15]  z1I=[1.4,-.2,.1;-.2,1.4,.1;.1,.1,2.25].*0  z2m=0  z2R=[1.4,0,.8]  z2I=[1.4,-.2,.1;-.2,1.4,.1;.1,.1,2.25].*0  z3m=0  z3R=[.75,-.5,.4]  z3I=[5,-.1,-2;-2,9,.1;-.1,.1,6].*0  z4m=0  z4R=[.75,.5,.4]  z4I=[5,-.1,-2;-2,9,.1;-.1,.1,6].*0  z5m=0  z5R=[1.25,-.5,.4]  z5I=[5,-.1,-2;-2,9,.1;-.1,.1,6].*0  z6m=0  z6R=[1.25,-.5,.4]  z6I=[5,-.1,-2;-2,9,.1;-.1,.1,6].*0  z7m=0  z7R=[2,0,.25]  z7I=[1.4,-.2,.1;-.2,1.4,.1;.1,.1,2.25].*0  Af=VEH.FrontalArea  Cd=.3  Cl=.1  Cpm=.1  beta_w=[0:0.01:0.3]  Cs=[0:0.03:0.9]  Cym=[0:0.01:0.3]  Pabs=101325  extTamb=off  Tair=273  g=9.81  xdot_tol=.1  longOff=0  latOff=0  vertOff=0.0112  wrapAng=off  aMode=2
  Vehicle1 : Outport
  wires:
  Vehicle Body 6DOF/5 -> Terminator9/1
  Suspension/1 -> Bus Selector3/1
  Vehicle Body 6DOF/2 -> Terminator6/1
  Ground1/1 -> Vehicle Body 6DOF/4
  Vehicle Body 6DOF/7 -> Terminator11/1
  Constant/1 -> Vehicle Body 6DOF/5
  Bus Selector3/2 -> Vehicle Body 6DOF/2  "<M>"
  Vehicle Body 6DOF/1 -> Vehicle1/1
  Bus Selector3/1 -> Vehicle Body 6DOF/1  "<F>"
  Vehicle Body 6DOF/6 -> Terminator10/1
  Vehicle Body 6DOF/4 -> Terminator8/1
  Vehicle Body 6DOF/3 -> Terminator7/1
  Ground/1 -> Vehicle Body 6DOF/3

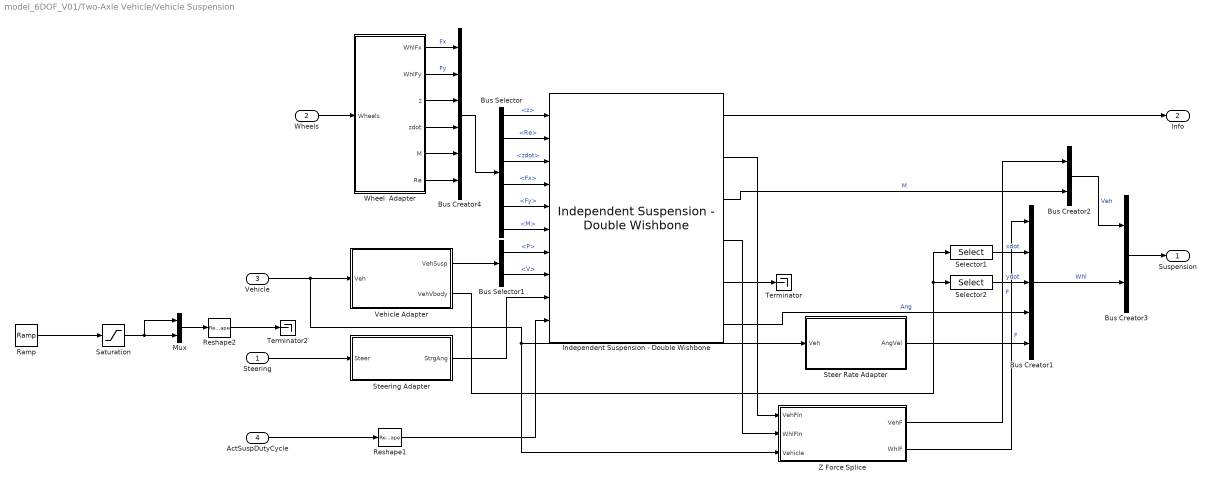
== system model_6DOF_V01/Two-Axle Vehicle/Vehicle Suspension ==
  Steering : Inport
  Wheels : Inport  Port=2
  Vehicle : Inport  Port=3
  ActSuspDutyCycle : Inport  Port=4
  Bus Creator1 : BusCreator  Inputs=5
  Bus Creator2 : BusCreator  Inputs=2
  Bus Creator3 : BusCreator  Inputs=2
  Bus Creator4 : BusCreator  Inputs=6
  Bus Selector : BusSelector  OutputSignals=z,Re,zdot,Fx,Fy,M
  Bus Selector1 : BusSelector  OutputSignals=P,V
  Independent Suspension - Double Wishbone : vehdynlibsuspension/Independent Suspension - Double Wishbone  ActiveDampEn=on  NumAxl=2  NumWhlsByAxl=[2 2]  StrgEnByAxl=[1 0]  AntiSwayEnByAxl=[0 0]  WhlNumVec="[1  2  1  2]"  AxleNumVec="[1  1  2  2]"  SuspTypesByAxle="[1  1]"  SuspImage=suspdw.png  IdealSuspEn=on  IdealSuspAxles="[1  2]"  Kz=64370  F0z=9810  Cz=10000  Hmax=0.5  f_act_susp_cz=[10000 10000;10000 10000]  f_act_susp_duty_bpt=[0 1]  f_act_susp_zdot_bpt=[-1 1]  Toe=0.0349  RollStrgSlp=-0.2269  ToeStrgSlp=0.01  Caster=0.0698  CasterHslp=-0.2269  CasterStrgSlp=0.01  Camber=0.0698  CamberHslp=-0.2269  CamberStrgSlp=0.01  StrgHgtSlp=0.1432  MappedSuspEn=off  MappedSuspAxles="[1  2]"  f_susp_axl_bp=[1 2]  f_susp_dz_bp=[-0.15 -0.14 -0.13 -0.12 -0.11 -0.10 -0.09 -0.08 -0.07 -0.06 -0.05 -0.04 -0.03 -0.02 -0.01 0.00 0.01 0.02 0.03 0.04 0.05 0.06 0.07 0.08 0.09 0.10 0.11 0.12 0.13 0.14 0.15]  f_susp_dzdot_bp=[-0.15 -0.14 -0.13 -0.12 -0.11 -0.10 -0.09 -0.08 -0.07 -0.06 -0.05 -0.04 -0.03 -0.02 -0.01 0.00 0.01 0.02 0.03 0.04 0.05 0.06 0.07 0.08 0.09 0.10 0.11 0.12 0.13 0.14 0.15]  f_susp_fmz=zeros(31,31,61,2,4)  f_susp_geom=zeros(31,61,2,3)  f_susp_strgdelta_bp=[-30,-29,-28,-27,-26,-25,-24,-23,-22,-21,-20,-19,-18,-17,-16,-15,-14,-13,-12,-11,-10,-9,-8,-7,-6,-5,-4,-3,-2,-1,0,1,2,3,4,5,6,7,8,9,10,11,12,13,14,15,16,17,18,19,20,21,22,23,24,25,26,27,28,29,30]  AntiSwayR=0.2  AntiSwayNtrlAng=0.5236  AntiSwayTrsK=5.7296e+03
      link override For each track and axle combination calculate suspension forces and moments/Suspension/Z axis suspension characteristic: LabelModeActiveChoice=IdealActiveSuspension
  Mux : Mux  Inputs=2
  Ramp : simulink/Sources/Ramp  slope=0.1  start=1  InitialOutput=0
  Reshape1 : Reshape  OutputDimensionality=Row vector (2-D)
  Reshape2 : Reshape  OutputDimensionality=Row vector (2-D)
  Saturation : Saturate
  Selector1 : Selector  NumberOfDimensions=2  InputPortWidth=3  IndexOptions=Index vector (dialog),Select all  Indices=1,1  OutputSizes=1,1
  Selector2 : Selector  NumberOfDimensions=2  InputPortWidth=3  IndexOptions=Index vector (dialog),Select all  Indices=2,1  OutputSizes=1,1
  Steer Rate Adapter : Subsystem
  Steering Adapter : Subsystem
  Terminator : Terminator
  Terminator2 : Terminator
  Vehicle Adapter : Subsystem
  Wheel  Adapter : Subsystem
  Z Force Splice : Subsystem  Variant=on  VariantControlMode=label  LabelModeActiveChoice=1
  Suspension : Outport
  Info : Outport  Port=2
  wires:
  Wheel  Adapter/6(Re) -> Bus Creator4/6
  Bus Selector1/1 -> Independent Suspension - Double Wishbone/7  "<P>"
  Bus Selector/6 -> Independent Suspension - Double Wishbone/6  "<M>"
  Bus Selector/1 -> Independent Suspension - Double Wishbone/1  "<z>"
  Bus Selector/5 -> Independent Suspension - Double Wishbone/5  "<Fy>"
  Wheel  Adapter/1(WhlFx) -> Bus Creator4/1  "Fx"
  Bus Selector/4 -> Independent Suspension - Double Wishbone/4  "<Fx>"
  Wheel  Adapter/4(zdot) -> Bus Creator4/4
  Wheel  Adapter/2(WhlFy) -> Bus Creator4/2  "Fy"
  Independent Suspension - Double Wishbone/1 -> Info/1
  Vehicle Adapter/1(VehSusp) -> Bus Selector1/1
  Bus Creator4/1 -> Bus Selector/1
  Bus Selector1/2 -> Independent Suspension - Double Wishbone/8  "<V>"
  Steering/1 -> Steering Adapter/1(Steer)
  Bus Selector/3 -> Independent Suspension - Double Wishbone/3  "<zdot>"
  Wheel  Adapter/3(z) -> Bus Creator4/3
  Wheel  Adapter/5(M) -> Bus Creator4/5
  Bus Selector/2 -> Independent Suspension - Double Wishbone/2  "<Re>"
  Vehicle Adapter/2(VehVbody) -> Selector1/1, Selector2/1
  Wheels/1 -> Wheel  Adapter/1(Wheels)
  Steering Adapter/1(StrgAng) -> Independent Suspension - Double Wishbone/9
  Vehicle/1 -> Vehicle Adapter/1(Veh), Z Force Splice/3(Vehicle), Steer Rate Adapter/1(Veh)
  Bus Creator3/1 -> Suspension/1
  Selector2/1 -> Bus Creator1/3  "ydot"
  Independent Suspension - Double Wishbone/4 -> Z Force Splice/2(WhlFIn)
  Bus Creator2/1 -> Bus Creator3/1  "Veh"
  Independent Suspension - Double Wishbone/3 -> Bus Creator2/2  "M"
  Selector1/1 -> Bus Creator1/2  "xdot"
  Independent Suspension - Double Wishbone/6 -> Bus Creator1/4  "Ang"
  Independent Suspension - Double Wishbone/2 -> Z Force Splice/1(VehFIn)
  Bus Creator1/1 -> Bus Creator3/2  "Whl"
  Steer Rate Adapter/1(AngVel) -> Bus Creator1/5
  Z Force Splice/1(VehF) -> Bus Creator2/1  "F"
  Z Force Splice/2(WhlF) -> Bus Creator1/1  "F"
  Independent Suspension - Double Wishbone/5 -> Terminator/1
  ActSuspDutyCycle/1 -> Reshape1/1
  Reshape1/1 -> Independent Suspension - Double Wishbone/10
  Ramp/1 -> Saturation/1
  Saturation/1 -> Mux/1, Mux/2
  Mux/1 -> Reshape2/1
  Reshape2/1 -> Terminator2/1

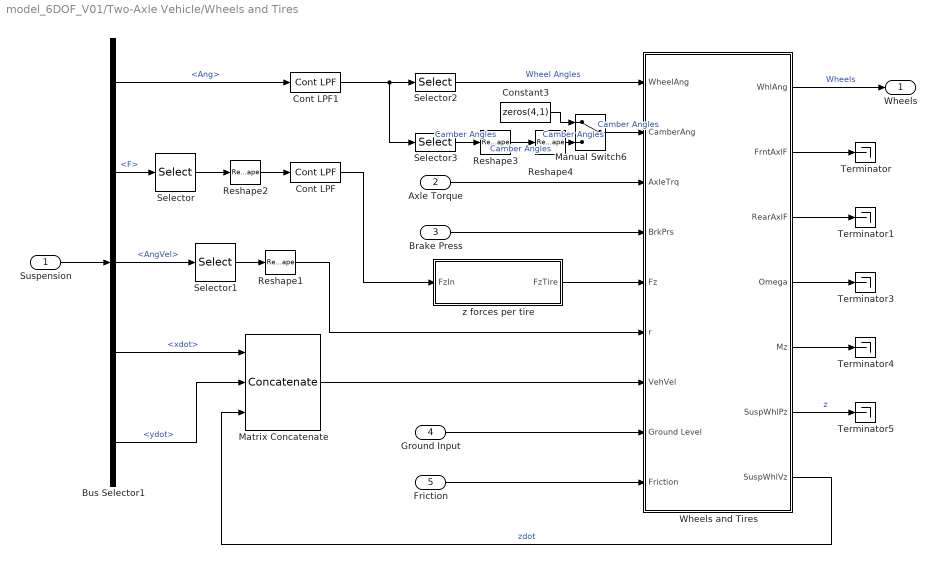
== system model_6DOF_V01/Two-Axle Vehicle/Wheels and Tires ==
  Suspension : Inport
  Axle Torque : Inport  Port=2
  Brake Press : Inport  Port=3  Unit=Pa
  Ground Input : Inport  Port=4
  Friction : Inport  Port=5
  Bus Selector1 : BusSelector  OutputSignals=Whl.Ang,Whl.F,Whl.AngVel,Whl.xdot,Whl.ydot
  Constant3 : Constant  Value=zeros(4,1)
  Cont LPF : autolibutils/Cont LPF  wc=100*2*pi  AbsoluteTolerance=auto  aMode=2
  Cont LPF1 : autolibutils/Cont LPF  wc=100*2*pi  AbsoluteTolerance=auto  aMode=2
  Manual Switch6 : ManualSwitch
  Matrix Concatenate : Concatenate  NumInputs=3  Mode=Multidimensional array
  Reshape1 : Reshape
  Reshape2 : Reshape
  Reshape3 : Reshape  OutputDimensionality=Column vector (2-D)
  Reshape4 : Reshape
  Selector : Selector  NumberOfDimensions=2  InputPortWidth=3  IndexOptions=Index vector (dialog),Select all  Indices=[3],1  OutputSizes=1,1
  Selector1 : Selector  NumberOfDimensions=2  InputPortWidth=1  IndexOptions=Index vector (dialog),Select all  Indices=[3],1  OutputSizes=1,1
  Selector2 : Selector  NumberOfDimensions=2  InputPortWidth=3  IndexOptions=Index vector (dialog),Select all  Indices=3,1  OutputSizes=1,1
  Selector3 : Selector  NumberOfDimensions=2  InputPortWidth=3  IndexOptions=Index vector (dialog),Select all  Indices=1,1  OutputSizes=1,1
  Terminator{,1,3..5} (5 alike) : Terminator
  Wheels and Tires : Subsystem  VariantControl=0
  z forces per tire : Subsystem
  Wheels : Outport  VectorParamsAs1DForOutWhenUnconnected=off
  wires:
  Wheels and Tires/1(WhlAng) -> Wheels/1  "Wheels"
  Bus Selector1/2 -> Selector/1  "<F>"
  Wheels and Tires/2(FrntAxlF) -> Terminator/1
  Wheels and Tires/3(RearAxlF) -> Terminator1/1
  Wheels and Tires/4(Omega) -> Terminator3/1
  Wheels and Tires/5(Mz) -> Terminator4/1
  Selector1/1 -> Reshape1/1
  Matrix Concatenate/1 -> Wheels and Tires/7(VehVel)
  Axle Torque/1 -> Wheels and Tires/3(AxleTrq)
  Selector2/1 -> Wheels and Tires/1(WheelAng)  "Wheel Angles"
  Constant3/1 -> Manual Switch6/1
  Manual Switch6/1 -> Wheels and Tires/2(CamberAng)  "Camber Angles"
  Selector/1 -> Reshape2/1
  z forces per tire/1(FzTire) -> Wheels and Tires/5(Fz)
  Ground Input/1 -> Wheels and Tires/8(Ground Level)
  Wheels and Tires/7(SuspWhlVz) -> Matrix Concatenate/3  "zdot"
  Bus Selector1/1 -> Cont LPF1/1  "<Ang>"
  Selector3/1 -> Reshape3/1  "Camber Angles"
  Suspension/1 -> Bus Selector1/1
  Bus Selector1/4 -> Matrix Concatenate/1  "<xdot>"
  Bus Selector1/5 -> Matrix Concatenate/2  "<ydot>"
  Wheels and Tires/6(SuspWhlPz) -> Terminator5/1  "z"
  Reshape2/1 -> Cont LPF/1
  Bus Selector1/3 -> Selector1/1  "<AngVel>"
  Reshape1/1 -> Wheels and Tires/6(r)
  Brake Press/1 -> Wheels and Tires/4(BrkPrs)
  Friction/1 -> Wheels and Tires/9(Friction)
  Cont LPF1/1 -> Selector3/1, Selector2/1
  Reshape3/1 -> Reshape4/1  "Camber Angles"
  Reshape4/1 -> Manual Switch6/2  "Camber Angles"
  Cont LPF/1 -> z forces per tire/1(FzIn)

== system model_6DOF_V01/Two-Axle Vehicle/Vehicle Suspension/Steer Rate Adapter ==
  Veh : Inport
  Add : Sum
  Bus Selector3 : BusSelector  OutputSignals=BdyFrm.Cg.AngVel.r
  Constant : Constant  Value=zeros(1,4)
  Matrix Concatenate : Concatenate  NumInputs=3  Mode=Multidimensional array
  Matrix Concatenate1 : Concatenate  NumInputs=3  Mode=Multidimensional array
  Mux : Mux
  Reshape2 : Reshape  OutputDimensionality=Row vector (2-D)
  Reshape3 : Reshape  OutputDimensionality=Row vector (2-D)
  Reshape4 : Reshape  OutputDimensionality=Row vector (2-D)
  SteerRates : Constant  Value=zeros(1,4)
  AngVel : Outport  VectorParamsAs1DForOutWhenUnconnected=off
  wires:
  Reshape2/1 -> Matrix Concatenate1/1, Matrix Concatenate1/3, Matrix Concatenate1/2
  Constant/1 -> Reshape3/1
  Mux/1 -> Reshape4/1
  Bus Selector3/1 -> Mux/3, Mux/4, Mux/2, Mux/1  "<r>"
  Matrix Concatenate/1 -> Add/2
  SteerRates/1 -> Reshape2/1
  Reshape4/1 -> Matrix Concatenate/3
  Reshape3/1 -> Matrix Concatenate/2, Matrix Concatenate/1
  Matrix Concatenate1/1 -> Add/1
  Veh/1 -> Bus Selector3/1
  Add/1 -> AngVel/1  "AngVel"

== system model_6DOF_V01/Two-Axle Vehicle/Vehicle Suspension/Steering Adapter ==
  Steer : Inport
  Reshape1 : Reshape  OutputDimensionality=Row vector (2-D)
  StrgAng : Outport  VectorParamsAs1DForOutWhenUnconnected=off
  wires:
  Reshape1/1 -> StrgAng/1
  Steer/1 -> Reshape1/1

== system model_6DOF_V01/Two-Axle Vehicle/Vehicle Suspension/Vehicle Adapter ==
  Veh : Inport
  Bus Creator3 : BusCreator  Inputs=2
  Bus Selector1 : BusSelector  OutputSignals=InertFrm.FrntAxl.Lft.Disp.X,InertFrm.FrntAxl.Lft.Disp.Y,InertFrm.FrntAxl.Lft.Disp.Z,InertFrm.FrntAxl.Rght.Disp.X,InertFrm.FrntAxl.Rght.Disp.Y,InertFrm.FrntAxl.Rght.Disp.Z,InertFrm.RearAxl.Lft.Disp.X,InertFrm.RearAxl.Lft.Disp.Y,InertFrm.RearAxl.Lft.Disp.Z,InertFrm.RearAxl.Rght.Disp.X,InertFrm.RearAxl.Rght.Disp.Y,InertFrm.RearAxl.Rght.Disp.Z
  Bus Selector2 : BusSelector  OutputSignals=BdyFrm.FrntAxl.Lft.Vel.xdot,BdyFrm.FrntAxl.Lft.Vel.ydot,BdyFrm.FrntAxl.Lft.Vel.zdot,BdyFrm.FrntAxl.Rght.Vel.xdot,BdyFrm.FrntAxl.Rght.Vel.ydot,BdyFrm.FrntAxl.Rght.Vel.zdot,BdyFrm.RearAxl.Lft.Vel.xdot,BdyFrm.RearAxl.Lft.Vel.ydot,BdyFrm.RearAxl.Lft.Vel.zdot,BdyFrm.RearAxl.Rght.Vel.xdot,BdyFrm.RearAxl.Rght.Vel.ydot,BdyFrm.RearAxl.Rght.Vel.zdot
  Bus Selector3 : BusSelector  OutputSignals=InertFrm.FrntAxl.Lft.Vel.Xdot,InertFrm.FrntAxl.Lft.Vel.Ydot,InertFrm.FrntAxl.Lft.Vel.Zdot,InertFrm.FrntAxl.Rght.Vel.Xdot,InertFrm.FrntAxl.Rght.Vel.Ydot,InertFrm.FrntAxl.Rght.Vel.Zdot,InertFrm.RearAxl.Lft.Vel.Xdot,InertFrm.RearAxl.Lft.Vel.Ydot,InertFrm.RearAxl.Lft.Vel.Zdot,InertFrm.RearAxl.Rght.Vel.Xdot,InertFrm.RearAxl.Rght.Vel.Ydot,InertFrm.RearAxl.Rght.Vel.Zdot
  Inertial Frame CG to Axle Offset : Constant  Value=[zeros(2,4);VEH.HeightCG*ones(1,4)]
  Mux1 : Mux  Inputs=12
  Mux2 : Mux  Inputs=12
  Mux3 : Mux  Inputs=12
  Reshape : Reshape  OutputDimensionality=Customize  OutputDimensions=[3,4]
  Reshape1 : Reshape  OutputDimensionality=Customize  OutputDimensions=[3,4]
  Reshape2 : Reshape  OutputDimensionality=Customize  OutputDimensions=[3,4]
  Sum : Sum  Inputs=|+-
  VehSusp : Outport  VectorParamsAs1DForOutWhenUnconnected=off
  VehVbody : Outport  Port=2  VectorParamsAs1DForOutWhenUnconnected=off
  wires:
  Veh/1 -> Bus Selector3/1, Bus Selector2/1, Bus Selector1/1
  Reshape2/1 -> VehVbody/1  "V"
  Bus Creator3/1 -> VehSusp/1  "Veh"
  Reshape/1 -> Sum/1
  Bus Selector1/1 -> Mux2/1  "<X>"
  Bus Selector1/2 -> Mux2/2  "<Y>"
  Bus Selector1/3 -> Mux2/3  "<Z>"
  Bus Selector1/4 -> Mux2/4  "<X>"
  Bus Selector1/5 -> Mux2/5  "<Y>"
  Bus Selector1/6 -> Mux2/6  "<Z>"
  Bus Selector1/7 -> Mux2/7  "<X>"
  Bus Selector1/8 -> Mux2/8  "<Y>"
  Bus Selector1/9 -> Mux2/9  "<Z>"
  Bus Selector1/10 -> Mux2/10  "<X>"
  Bus Selector1/11 -> Mux2/11  "<Y>"
  Bus Selector1/12 -> Mux2/12  "<Z>"
  Bus Selector2/1 -> Mux1/1  "<xdot>"
  Bus Selector2/2 -> Mux1/2  "<ydot>"
  Bus Selector2/3 -> Mux1/3  "<zdot>"
  Bus Selector2/4 -> Mux1/4  "<xdot>"
  Bus Selector2/5 -> Mux1/5  "<ydot>"
  Bus Selector2/6 -> Mux1/6  "<zdot>"
  Bus Selector2/7 -> Mux1/7  "<xdot>"
  Bus Selector2/8 -> Mux1/8  "<ydot>"
  Bus Selector2/9 -> Mux1/9  "<zdot>"
  Bus Selector2/10 -> Mux1/10  "<xdot>"
  Bus Selector2/11 -> Mux1/11  "<ydot>"
  Bus Selector2/12 -> Mux1/12  "<zdot>"
  Mux1/1 -> Reshape2/1
  Mux2/1 -> Reshape/1
  Inertial Frame CG to Axle Offset/1 -> Sum/2
  Sum/1 -> Bus Creator3/1  "P"
  Mux3/1 -> Reshape1/1
  Bus Selector3/12 -> Mux3/12  "<Zdot>"
  Bus Selector3/11 -> Mux3/11  "<Ydot>"
  Bus Selector3/10 -> Mux3/10  "<Xdot>"
  Bus Selector3/9 -> Mux3/9  "<Zdot>"
  Bus Selector3/8 -> Mux3/8  "<Ydot>"
  Bus Selector3/7 -> Mux3/7  "<Xdot>"
  Bus Selector3/6 -> Mux3/6  "<Zdot>"
  Bus Selector3/5 -> Mux3/5  "<Ydot>"
  Bus Selector3/4 -> Mux3/4  "<Xdot>"
  Bus Selector3/3 -> Mux3/3  "<Zdot>"
  Bus Selector3/2 -> Mux3/2  "<Ydot>"
  Bus Selector3/1 -> Mux3/1  "<Xdot>"
  Reshape1/1 -> Bus Creator3/2  "V"

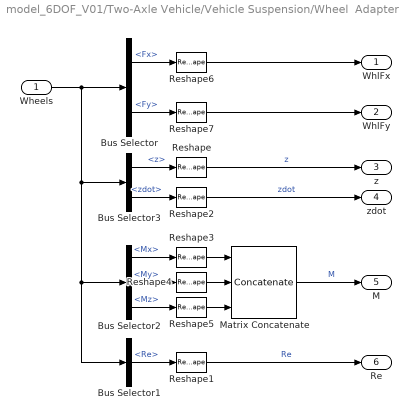
== system model_6DOF_V01/Two-Axle Vehicle/Vehicle Suspension/Wheel  Adapter ==
  Wheels : Inport
  Bus Selector : BusSelector  OutputSignals=TireFrame.Fx,TireFrame.Fy
  Bus Selector1 : BusSelector  OutputSignals=TireFrame.Re
  Bus Selector2 : BusSelector  OutputSignals=TireFrame.Mx,TireFrame.My,TireFrame.Mz
  Bus Selector3 : BusSelector  OutputSignals=TireFrame.z,TireFrame.zdot
  Matrix Concatenate : Concatenate  NumInputs=3  Mode=Multidimensional array
  Reshape{,1..7} (8 alike) : Reshape  OutputDimensionality=Row vector (2-D)
  WhlFx : Outport  VectorParamsAs1DForOutWhenUnconnected=off
  WhlFy : Outport  Port=2  VectorParamsAs1DForOutWhenUnconnected=off
  z : Outport  Port=3  VectorParamsAs1DForOutWhenUnconnected=off
  zdot : Outport  Port=4  VectorParamsAs1DForOutWhenUnconnected=off
  M : Outport  Port=5  VectorParamsAs1DForOutWhenUnconnected=off
  Re : Outport  Port=6  VectorParamsAs1DForOutWhenUnconnected=off
  wires:
  Reshape7/1 -> WhlFy/1
  Reshape6/1 -> WhlFx/1
  Bus Selector/1 -> Reshape6/1  "<Fx>"
  Bus Selector/2 -> Reshape7/1  "<Fy>"
  Bus Selector3/1 -> Reshape/1  "<z>"
  Wheels/1 -> Bus Selector1/1, Bus Selector2/1, Bus Selector3/1, Bus Selector/1
  Bus Selector3/2 -> Reshape2/1  "<zdot>"
  Reshape2/1 -> zdot/1  "zdot"
  Bus Selector1/1 -> Reshape1/1  "<Re>"
  Reshape1/1 -> Re/1  "Re"
  Bus Selector2/1 -> Reshape3/1  "<Mx>"
  Bus Selector2/2 -> Reshape4/1  "<My>"
  Bus Selector2/3 -> Reshape5/1  "<Mz>"
  Reshape3/1 -> Matrix Concatenate/1
  Reshape4/1 -> Matrix Concatenate/2
  Reshape5/1 -> Matrix Concatenate/3
  Matrix Concatenate/1 -> M/1  "M"
  Reshape/1 -> z/1  "z"

== system model_6DOF_V01/Two-Axle Vehicle/Vehicle Suspension/Z Force Splice ==
  note: 1) Add Subsystem or Model blocks as valid variant choices.
      | 2) You cannot connect blocks at this level. At simulation, connectivity is automatically
      | determined, based on the active variant and port name matching.
  VehFIn : Inport
  WhlFIn : Inport  Port=2
  Vehicle : Inport  Port=3
  Z Force Pass Through 6DOF : Subsystem  VariantControl=1
  Z Force Splice 3DOF : Subsystem  VariantControl=0
  VehF : Outport
  WhlF : Outport  Port=2

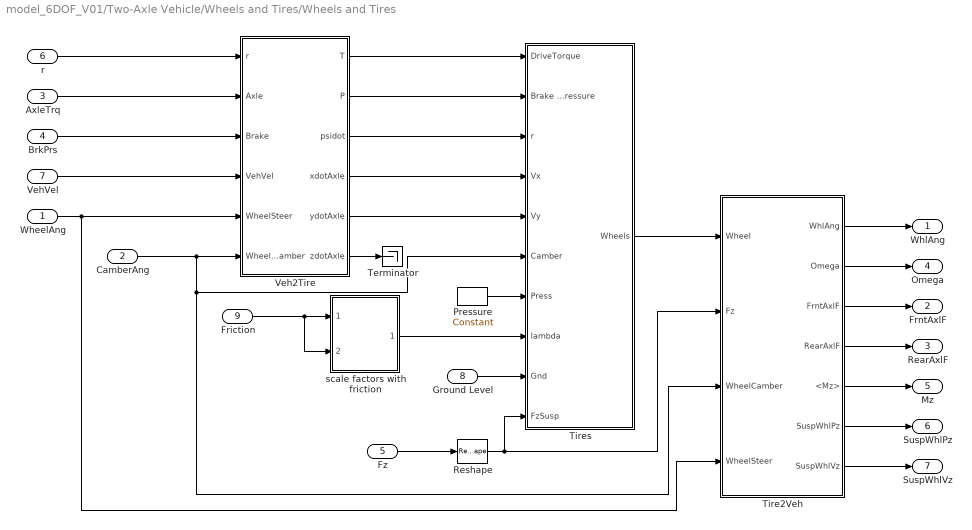
== system model_6DOF_V01/Two-Axle Vehicle/Wheels and Tires/Wheels and Tires ==
  WheelAng : Inport
  CamberAng : Inport  Port=2  Unit=rad
  AxleTrq : Inport  Port=3
  BrkPrs : Inport  Port=4
  Fz : Inport  Port=5  Unit=N
  r : Inport  Port=6
  VehVel : Inport  Port=7
  Ground Level : Inport  Port=8
  Friction : Inport  Port=9  Unit=1
  Pressure : vehdynlibtirecommon/Constant  const=220000  numWheels=4
  Reshape : Reshape
  Terminator : Terminator
  Tire2Veh : Subsystem
  Tires : Subsystem  Variant=on  VariantControlMode=label  VariantControl=Variant1  LabelModeActiveChoice=0
  Veh2Tire : Subsystem
  scale factors with friction : Subsystem  mask{numWheels=6}
      mask prompts: numWheels "Number of wheels"
  WhlAng : Outport  VectorParamsAs1DForOutWhenUnconnected=off
  FrntAxlF : Outport  Port=2  Unit=N  VectorParamsAs1DForOutWhenUnconnected=off
  RearAxlF : Outport  Port=3  Unit=N  VectorParamsAs1DForOutWhenUnconnected=off
  Omega : Outport  Port=4  VectorParamsAs1DForOutWhenUnconnected=off
  Mz : Outport  Port=5  Unit=N*m  VectorParamsAs1DForOutWhenUnconnected=off
  SuspWhlPz : Outport  Port=6  VectorParamsAs1DForOutWhenUnconnected=off
  SuspWhlVz : Outport  Port=7  VectorParamsAs1DForOutWhenUnconnected=off
  wires:
  Ground Level/1 -> Tires/9("Gnd ")
  Pressure/1 -> Tires/7("Press ")
  scale factors with friction/1(lambdas) -> Tires/8("lambda ")
  Fz/1 -> Reshape/1
  AxleTrq/1 -> Veh2Tire/2(Axle)
  BrkPrs/1 -> Veh2Tire/3(Brake)
  VehVel/1 -> Veh2Tire/4(VehVel)
  Veh2Tire/1(T) -> Tires/1("DriveTorque ")
  Veh2Tire/2(P) -> Tires/2("Brake Pressure ")
  Veh2Tire/4(xdotAxle) -> Tires/4("Vx ")
  Veh2Tire/5(ydotAxle) -> Tires/5("Vy ")
  Veh2Tire/3(psidot) -> Tires/3("r ")
  Tires/1(" Wheels") -> Tire2Veh/1(Wheel)
  WheelAng/1 -> Veh2Tire/5(WheelSteer), Tire2Veh/4(WheelSteer)
  Tire2Veh/2(Omega) -> Omega/1
  Tire2Veh/3(FrntAxlF) -> FrntAxlF/1
  Tire2Veh/5(<Mz>) -> Mz/1
  Friction/1 -> scale factors with friction/2(lamda_mu_y), scale factors with friction/1(lamda_mu_x)
  r/1 -> Veh2Tire/1(r)
  Veh2Tire/6(zdotAxle) -> Terminator/1
  Tire2Veh/6(SuspWhlPz) -> SuspWhlPz/1
  Tire2Veh/7(SuspWhlVz) -> SuspWhlVz/1
  CamberAng/1 -> Tires/6("Camber "), Tire2Veh/3(WheelCamber), Veh2Tire/6(WheelCamber)
  Tire2Veh/1(WhlAng) -> WhlAng/1
  Tire2Veh/4(RearAxlF) -> RearAxlF/1
  Reshape/1 -> Tire2Veh/2(Fz), Tires/10("FzSusp ")

== system model_6DOF_V01/Two-Axle Vehicle/Wheels and Tires/z forces per tire ==
  FzIn : Inport
  Demux : Demux
  Gain12 : Gain  Gain=1/VEH.NumberOfWheelsPerRearAxle
  Gain13 : Gain  Gain=1/VEH.NumberOfWheelsPerRearAxle
  Gain14 : Gain  Gain=2
  Gain8 : Gain  Gain=1/VEH.NumberOfWheelsPerFrontAxle
  Gain9 : Gain  Gain=1/VEH.NumberOfWheelsPerFrontAxle
  Mux1 : Mux
  FzTire : Outport
  wires:
  Demux/2 -> Gain9/1
  Gain14/1 -> FzTire/1
  Gain8/1 -> Mux1/1
  Mux1/1 -> Gain14/1
  Gain9/1 -> Mux1/2
  Demux/1 -> Gain8/1
  FzIn/1 -> Demux/1
  Demux/3 -> Gain12/1
  Gain12/1 -> Mux1/3
  Gain13/1 -> Mux1/4
  Demux/4 -> Gain13/1

== system model_6DOF_V01/Two-Axle Vehicle/Vehicle Suspension/Z Force Splice/Z Force Pass Through 6DOF ==
  VehFIn : Inport
  WhlFIn : Inport  Port=2
  Vehicle : Inport  Port=3
  Terminator : Terminator
  VehF : Outport
  WhlF : Outport  Port=2
  wires:
  VehFIn/1 -> VehF/1  "F"
  WhlFIn/1 -> WhlF/1  "F"
  Vehicle/1 -> Terminator/1

== system model_6DOF_V01/Two-Axle Vehicle/Vehicle Suspension/Z Force Splice/Z Force Splice 3DOF ==
  VehFIn : Inport
  WhlFIn : Inport  Port=2
  Vehicle : Inport  Port=3
  Bus Selector2 : BusSelector  OutputSignals=BdyFrm.Forces.Tires.FrntTires.Lft.Fz,BdyFrm.Forces.Tires.FrntTires.Rght.Fz,BdyFrm.Forces.Tires.RearTires.Lft.Fz,BdyFrm.Forces.Tires.RearTires.Rght.Fz
  Constant : Constant  Value=VEH.Mass*9.81/4
  Cont LPF IC : autolibutils/Cont LPF IC  wc=1/0.01  aMode=2  dataType=off
  Gain : Gain  Gain=-1
  Gain1 : Gain  Gain=VEH.NumberOfWheelsPerFrontAxle
  Gain2 : Gain  Gain=VEH.NumberOfWheelsPerFrontAxle
  Gain5 : Gain  Gain=VEH.NumberOfWheelsPerRearAxle
  Gain6 : Gain  Gain=VEH.NumberOfWheelsPerRearAxle
  Gain7 : Gain  Gain=1/2
  Matrix Concatenate : Concatenate  Mode=Multidimensional array
  Matrix Concatenate1 : Concatenate  Mode=Multidimensional array
  Mux : Mux
  Reshape : Reshape  OutputDimensionality=Row vector (2-D)
  Selector4 : Selector  NumberOfDimensions=2  InputPortWidth=3  IndexOptions=Index vector (dialog),Select all  Indices=[1 2],1  OutputSizes=1,1
  Selector5 : Selector  NumberOfDimensions=2  InputPortWidth=3  IndexOptions=Index vector (dialog),Select all  Indices=[1 2],1  OutputSizes=1,1
  VehF : Outport
  WhlF : Outport  Port=2
  wires:
  Vehicle/1 -> Bus Selector2/1
  Bus Selector2/4 -> Gain6/1  "<Fz>"
  Selector5/1 -> Matrix Concatenate1/1
  Gain5/1 -> Mux/3
  Constant/1 -> Cont LPF IC/2
  Matrix Concatenate/1 -> WhlF/1  "F"
  Gain1/1 -> Mux/1
  Gain7/1 -> Cont LPF IC/1
  Cont LPF IC/1 -> Reshape/1
  Gain/1 -> Matrix Concatenate1/2
  Gain2/1 -> Mux/2
  Reshape/1 -> Gain/1, Matrix Concatenate/2
  VehFIn/1 -> Selector5/1
  Selector4/1 -> Matrix Concatenate/1
  Bus Selector2/3 -> Gain5/1  "<Fz>"
  Bus Selector2/1 -> Gain1/1  "<Fz>"
  Matrix Concatenate1/1 -> VehF/1  "F"
  Mux/1 -> Gain7/1
  WhlFIn/1 -> Selector4/1
  Gain6/1 -> Mux/4
  Bus Selector2/2 -> Gain2/1  "<Fz>"
